simulink model "rotpen_MPC_poly"  (R2025b)
settings: Solver=ode45  StartTime=0.0  StopTime=60  RelTol=1e-3  EnableMultiTasking=on
values from neighbouring files (symbols this model uses):
  A_ineq = A_block * Su    [MPC_poly.m]
  b_ineq_base = b_block    [MPC_poly.m]
  F_qp = 2 * Su' * Q_bar * Sx    [MPC_poly.m]
  h = 0.01    [MPC.m]    (also in MPC_poly.m = 0.05; Robus_controller.m; data_ext.m)
  H_qp = (H_qp + H_qp') / 2    [MPC_poly.m]
  N = 20    [MPC.m]    (also in MPC_poly.m = 5)
  n_states = 4    [MPC.m]    (also in MPC_poly.m)
  R2 = diag([1e-2, 1e-2])    [MPC_poly.m]    (also in state_est.m = diag([1e-1, 1e-1]))
  S_ineq = A_block * Sx    [MPC_poly.m]
  u_max = 2.0    (= 2)    [MPC.m]    (also in MPC_poly.m)
undefined symbols (not defined in the file or in its folder): adingain, adinoffs, daoutgain, daoutoffs, Discrete, Time
libraries: ctrlSharedLib x1
settings Model: Creator=rbabuska  LastModifiedBy=root
settings SolverCC: AlgebraicLoopSolver=TrustRegion
settings DataIOCC: LimitDataPoints=on  SaveFormat=Array  ReturnWorkspaceOutputs=off  SignalLoggingName=sigsOut
settings OptimizationCC: BooleanDataType=off  ExpressionDepthLimit=2147483647.0  InitFltsAndDblsToZero=on  LifeSpan=inf
settings DebuggingCC: SaveWithParameterizedLinksMsg=none  SignalResolutionControl=TryResolveAllWithWarning  MultiTaskDSMMsg=warning  MultiTaskCondExecSysMsg=none  UnconnectedInputMsg=warning  UnconnectedOutputMsg=warning  UnconnectedLineMsg=warning  AllowSymbolicDim=off  StateNameClashWarn=warning  SFUnexpectedBacktrackingDiag=warning  SFNoUnconditionalDefaultTransitionDiag=warning  SFExecutionAtInitializationDiag=none  ArithmeticOperatorsInVariantConditions=warning
settings HardwareCC: ProdBitPerPointer=32.0  ProdBitPerSizeT=32.0  ProdBitPerPtrDiffT=32.0  ProdLargestAtomicFloat=None  ProdIntDivRoundTo=Undefined  ProdEndianess=Unspecified  ProdWordSize=32.0  ProdHWDeviceType=32-bit Generic  TargetBitPerLong=64.0  TargetBitPerPointer=64.0  TargetBitPerSizeT=64.0  TargetBitPerPtrDiffT=64.0  TargetLongLongMode=on  TargetIntDivRoundTo=Zero  TargetEndianess=LittleEndian  TargetWordSize=64.0  TargetHWDeviceType=MATLAB Host  ProdEqTarget=off
settings ModelReferenceCC: EnableRefExpFcnMdlSchedulingChecks=on  PropagateSignalLabelsOutOfModel=off
settings SFSimCC: SimUseLocalCustomCode=off  CustomCodeUndefinedFunction=UseInterfaceOnly
settings RTWCC: RTWUseLocalCustomCode=off  GPUComputeCapability=3.5  DLArmComputeVersion=19.05
settings CodeAppCC: StateflowObjectComments=on
settings GRTTargetCC: TargetFcnLib=ansi_tfl_tmw.mat  TargetLangStandard=C89/C90 (ANSI)  CombineOutputUpdateFcns=off  GRTInterface=on
settings ConfigComp: CovMetricSettings=dw  CovSaveCumulativeToWorkspaceVar=on  CovSaveSingleToWorkspaceVar=on  CovExternalEMLEnable=off

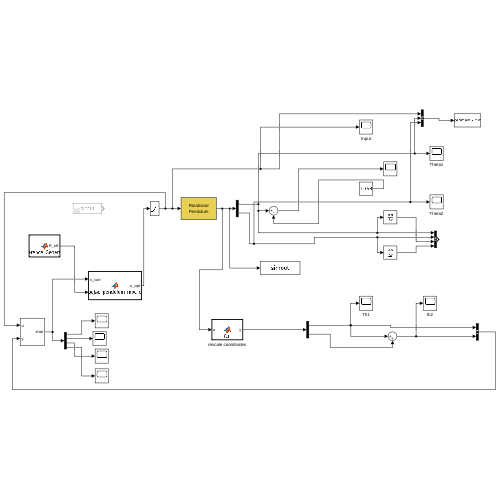
[thumbnail: Simulink's stored preview of the top-level diagram]
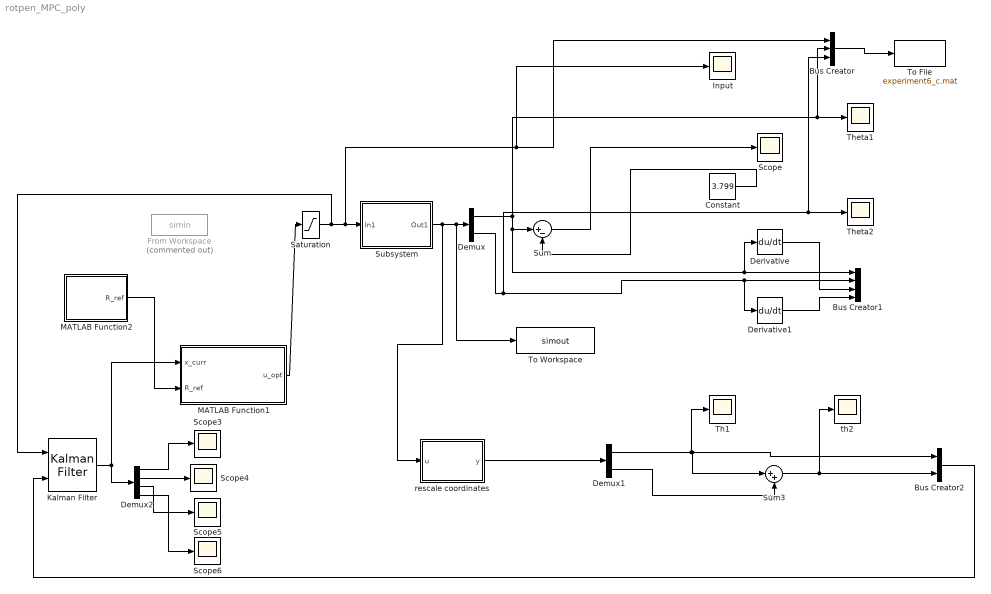
== system rotpen_MPC_poly ==
  Bus Creator : BusCreator  Inputs=3
  Bus Creator1 : BusCreator  Inputs=4
  Bus Creator2 : BusCreator  Inputs=2
  Constant : Constant  Value=3.799
  Demux : Demux  Outputs=2
  Demux1 : Demux  Outputs=2
  Demux2 : Demux
  Derivative : Derivative
  Derivative1 : Derivative
  From Workspace : FromWorkspace  Commented=on  VariableName=simin
  Input : Scope
      settings: ActiveDisplayYMinimum=-1.25  ActiveDisplayYMaximum=1.25
  Kalman Filter : ctrlSharedLib/Kalman Filter  TimeDomain=Discrete-Time  UseCurrentEstimator=on  ModelSource=LTI State-Space Variable  ModelSourceVariable=sysd  A=0.95  B=1  C=1  D=0  NumberOfStates=1  NumberOfInputs=1  NumberOfOutputs=1  InitialEstimateSource=Dialog  X0=0  P0=10  UseK=off  UseGH=off  NumberOfProcessNoiseInputs=1  G=1  TimeInvariantG=on  H=0  TimeInvariantH=on  Q=R1  TimeInvariantQ=on  R=R2  TimeInvariantR=on  N=0  TimeInvariantN=on  AddInputPort=on  AddEnablePort=off  OutputEstimatedY=off  OutputP=off  Ts=-1
  MATLAB Function1 : MATLAB Function  TreatAsAtomicUnit=on
  MATLAB Function2 : MATLAB Function  TreatAsAtomicUnit=on
  Saturation : Saturate  UpperLimit=1  LowerLimit=-1
  Scope{,3..6} (5 alike) : Scope
      Scope settings: ActiveDisplayYMinimum=-4.4086  ActiveDisplayYMaximum=1.6874
      Scope3 settings: ActiveDisplayYMinimum=-3.524  ActiveDisplayYMaximum=3.8049
      Scope4 settings: ActiveDisplayYMinimum=-4.6221  ActiveDisplayYMaximum=4.3572  DataLoggingVariableName=ScopeData2
      Scope5 settings: ActiveDisplayYMinimum=-1.3955  ActiveDisplayYMaximum=1.6015  DataLoggingVariableName=ScopeData3
      Scope6 settings: ActiveDisplayYMinimum=-0.94416  ActiveDisplayYMaximum=0.81176  DataLoggingVariableName=ScopeData4
  Subsystem : Subsystem
      mask Display: disp('Rotational\nPendulum')
  Sum : Sum  Inputs=|+-
  Sum3 : Sum  Inputs=|++
  Th1 : Scope
      settings: ActiveDisplayYMinimum=-3.9253  ActiveDisplayYMaximum=3.9267  DataLoggingVariableName=ScopeData2
  Theta1 : Scope
      settings: ActiveDisplayYMinimum=-0.61128  ActiveDisplayYMaximum=5.5015
  Theta2 : Scope
      settings: ActiveDisplayYMinimum=-0.61799  ActiveDisplayYMaximum=5.5619  DataLoggingVariableName=ScopeData2
  To File : ToFile  Filename=experiment6_c.mat
  To Workspace : ToWorkspace  VariableName=simout  SaveFormat=Timeseries  SampleTime=-1
  rescale coordinates : MATLAB Function  TreatAsAtomicUnit=on
  th2 : Scope
      settings: ActiveDisplayYMinimum=-5.7167  ActiveDisplayYMaximum=6.5045  DataLoggingVariableName=ScopeData3
  wires:
  Demux/1 -> Sum/1, Derivative/1, Bus Creator1/1, Bus Creator/2, Theta1/1
  Demux/2 -> Theta2/1, Bus Creator/3, Derivative1/1, Bus Creator1/2
  Bus Creator/1 -> To File/1
  Derivative/1 -> Bus Creator1/3
  Derivative1/1 -> Bus Creator1/4
  Constant/1 -> Sum/2
  Sum/1 -> Scope/1
  Kalman Filter/1 -> MATLAB Function1/1(x_curr), Demux2/1
  Bus Creator2/1 -> Kalman Filter/2
  Demux1/2 -> Sum3/2
  Subsystem/1(Out1) -> rescale coordinates/1(u), To Workspace/1, Demux/1
  Saturation/1 -> Kalman Filter/1, Subsystem/1(In1), Bus Creator/1, Input/1
  Sum3/1 -> th2/1, Bus Creator2/2
  Demux1/1 -> Bus Creator2/1, Sum3/1, Th1/1
  Demux2/1 -> Scope3/1
  Demux2/4 -> Scope6/1
  Demux2/3 -> Scope5/1
  Demux2/2 -> Scope4/1
  rescale coordinates/1(y) -> Demux1/1
  MATLAB Function1/1(u_opt) -> Saturation/1
  MATLAB Function2/1(R_ref) -> MATLAB Function1/2(R_ref)

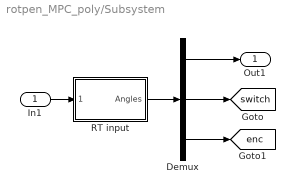
== system rotpen_MPC_poly/Subsystem ==
  In1 : Inport
  Demux : Demux  Outputs=[2 4 1]
  RT input : Subsystem  mask{Ts=h, channels=[6 7]}
      mask prompts: Ts "Sample time [s]:"; channels "Channels to read (e.g., [6 7])"
      mask init:
      | hwinit;
      | 
      | % initialize FPGA
      | fugihandle = fugiboard('Open', 'Pendulum1');
      | fugihandle.WatchdogTimeout = 0.5;
      | fugiboard('SetParams', fugihandle);
      | fugiboard('Write', fugihandle, 0, 0, 0, 0);  % dummy write to sync interface board
      | fugiboard('Write', fugihandle, 5, 1, 0, 0);  % reset position, activate relay
      | data = fugiboard('Read', fugihandle);        % get version info from FPGA
      | % model = bitshift(data(1), -5); 
      | % version = bitand(data(1), 31);
      | % disp(sprintf('FPGA setup %d, version %d', model, version)); % for the B&P it should say 1 1, or else there is a problem
      | fugiboard('Write', fugihandle, 0, 1, 0, 0);  % end reset
      | pause(0.1);                         % give relay some time to respond
      mask Display: disp('Rotational\nPendulum')
  Out1 : Outport
  tag scope: enc=global, switch=global
  wires:
  RT input/1(Angles) -> Demux/1
  Demux/1 -> Out1/1
  Demux/2 -> [switch]
  Demux/3 -> [enc]
  In1/1 -> RT input/1(Motors)

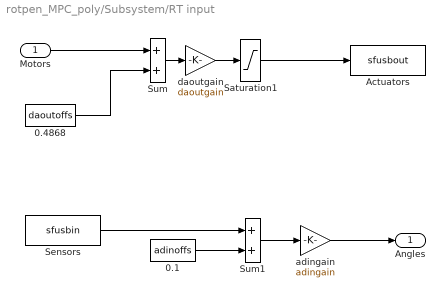
== system rotpen_MPC_poly/Subsystem/RT input ==
  Motors : Inport
  0.1 : Constant  Value=adinoffs
  0.4868 : Constant  Value=daoutoffs
  Actuators : S-Function  FunctionName=sfusbout  Parameters=Ts, fugihandle  SFunctionDeploymentMode=off  EnableBusSupport=off
  Saturation1 : Saturate  UpperLimit=10  LowerLimit=-10
  Sensors : S-Function  FunctionName=sfusbin  Parameters=Ts, fugihandle, channels  SFunctionDeploymentMode=off  EnableBusSupport=off
  Sum : Sum  InputSameDT=on  SaturateOnIntegerOverflow=on  OutDataTypeStr=Inherit: Same as first input
  Sum1 : Sum  InputSameDT=on  SaturateOnIntegerOverflow=on  OutDataTypeStr=Inherit: Same as first input
  adingain : Gain  Gain=adingain  SaturateOnIntegerOverflow=on  OutDataTypeStr=Inherit: Same as input  ParamDataTypeStr=Inherit: Same as input
  daoutgain : Gain  Gain=daoutgain  SaturateOnIntegerOverflow=on  OutDataTypeStr=Inherit: Same as input  ParamDataTypeStr=Inherit: Same as input
  Angles : Outport
  wires:
  Sum/1 -> daoutgain/1
  0.4868/1 -> Sum/2
  Motors/1 -> Sum/1
  Sum1/1 -> adingain/1
  0.1/1 -> Sum1/2
  adingain/1 -> Angles/1
  Saturation1/1 -> Actuators/1
  daoutgain/1 -> Saturation1/1
  Sensors/1 -> Sum1/1

== matlab function rotpen_MPC_poly/rescale coordinates ==
  data: u input; y output
function y = fcn(u)
th1in = u(1);
th2in = u(2);

scale1 = 4.881666285191120;
scale2 = 4.932936598764020;

% eq1 = 3.796622000341846/scale1 *2*pi;
% eq2 = 1.210150569834988/scale2 *2*pi+pi;
%down up
% eq1 = 3.806622000341846/scale1 *2*pi;
% eq2 = 1.189150569834988/scale2 *2*pi + pi + 2*pi/360*7.5;

%up up
eq1 = 3.806622000341846/scale1 *2*pi+ pi - 2*pi/360*14;
eq2 = 1.189150569834988/scale2 *2*pi + 2*pi/360*5;


th1 = mod(th1in/scale1*2*pi - eq1 +pi, 2*pi) -pi;
th2 = mod(th2in/scale2*2*pi - eq2 +pi, 2*pi) -pi;

y = [th1
     th2];

== matlab function rotpen_MPC_poly/MATLAB Function1 ==
  data: x_curr input; u_opt output; H_qp parameter; F_qp parameter; A_ineq parameter; b_ineq_base parameter; S_ineq parameter; N parameter; u_max parameter; R_ref input
function u_opt = double_pendulum_mpc_qp(x_curr, H_qp, F_qp, A_ineq, b_ineq_base, S_ineq, N, u_max, R_ref)
    
    % 1. Calculate state-dependent linear objective
    f = F_qp * x_curr + F_ref * R_ref;
    
    % 2. Calculate state-dependent constraint boundaries
    b_ineq = b_ineq_base - S_ineq * x_curr;
    
    r_N = R_ref((N-1)*n_states+1 : N*n_states);

    % 3. Define Input Bounds (Constraints on U directly)
    lb = -u_max * ones(N, 1);
    ub =  u_max * ones(N, 1);

    m_poly = size(H_poly, 1);
    b_ineq(end-m_poly+1 : end) = b_ineq(end-m_poly+1 : end) + H_poly * r_N;
    
    % 4. Solve QP
    options = optimoptions('quadprog', 'Display', 'none', 'Algorithm', 'active-set');
    
    % quadprog signature: x = quadprog(H, f, A, b, Aeq, beq, lb, ub, x0, options)
    [U_opt, ~, exitflag] = quadprog(H_qp, f, A_ineq, b_ineq, [], [], lb, ub, [], options);
        
    % 5. Handle output
    if exitflag <= 0
        u_opt = 0; % Fallback if solver fails (e.g., infeasible)
    else
        u_opt = U_opt(1); % Apply only the first optimal control action
    end
end

== matlab function rotpen_MPC_poly/MATLAB Function2 ==
  data: R_ref output; N parameter; h parameter; n_states parameter; t data_store_memory
function R_ref = Reference_Generator(N, h, n_states)
    %#codegen
    % t: current simulation time (seconds)
    % signal_type: 1 for Sine, 2 for Block/Square
    % amplitude: scaling factor
    % frequency: in Hz
    % h: sample time (0.05s)
    
    R_ref = zeros(N * n_states, 1);
    
    for k = 1:N
        % Calculate the absolute future time for this horizon step
        t_future = t + k * h;
        
        r_val = Reference(t_future);
        
        % Map the scalar reference to your target state vector 
        % Assuming we are tracking a position target on Theta 1: [theta1; 0; 0; 0]
        x_ref_k = [r_val; 0; 0; 0];
        
        % Assign to the stacked R_ref vector
        idx_start = (k-1) * n_states + 1;
        idx_end = k * n_states;
        R_ref(idx_start:idx_end) = x_ref_k;
    end
end


function r_val = Reference(t)

    r_val = 0.3 * sin(2 * pi * 1/5 * t);
end
